simulink model "PthSet"  (R2018a)
settings: configuration reference "cs_ert" (kept outside this file)
settings Model: DataDictionary=PthSet.sldd  Creator=zhoutinglin  LastModifiedBy=zhoutinglin

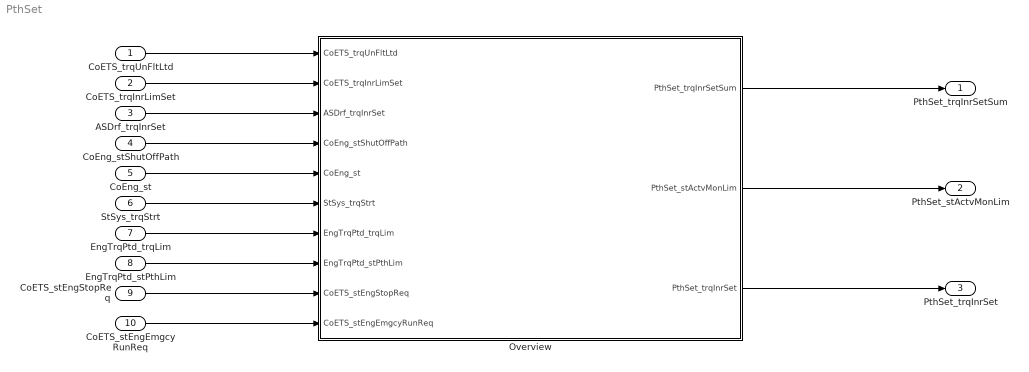
== system PthSet ==
  CoETS_trqUnFltLtd : Inport
  CoETS_trqInrLimSet : Inport  Port=2
  ASDrf_trqInrSet : Inport  Port=3
  CoEng_stShutOffPath : Inport  Port=4
  CoEng_st : Inport  Port=5
  StSys_trqStrt : Inport  Port=6
  EngTrqPtd_trqLim : Inport  Port=7
  EngTrqPtd_stPthLim : Inport  Port=8
  CoETS_stEngStopReq : Inport  Port=9
  CoETS_stEngEmgcyRunReq : Inport  Port=10
  Overview : Subsystem
  PthSet_trqInrSetSum : Outport
  PthSet_stActvMonLim : Outport  Port=2
  PthSet_trqInrSet : Outport  Port=3
  wires:
  CoETS_trqUnFltLtd/1 -> Overview/1(CoETS_trqUnFltLtd)
  CoETS_trqInrLimSet/1 -> Overview/2(CoETS_trqInrLimSet)
  ASDrf_trqInrSet/1 -> Overview/3(ASDrf_trqInrSet)
  CoEng_stShutOffPath/1 -> Overview/4(CoEng_stShutOffPath)
  CoEng_st/1 -> Overview/5(CoEng_st)
  StSys_trqStrt/1 -> Overview/6(StSys_trqStrt)
  EngTrqPtd_trqLim/1 -> Overview/7(EngTrqPtd_trqLim)
  EngTrqPtd_stPthLim/1 -> Overview/8(EngTrqPtd_stPthLim)
  CoETS_stEngStopReq/1 -> Overview/9(CoETS_stEngStopReq)
  CoETS_stEngEmgcyRunReq/1 -> Overview/10(CoETS_stEngEmgcyRunReq)
  Overview/1(PthSet_trqInrSetSum) -> PthSet_trqInrSetSum/1
  Overview/2(PthSet_stActvMonLim) -> PthSet_stActvMonLim/1
  Overview/3(PthSet_trqInrSet) -> PthSet_trqInrSet/1

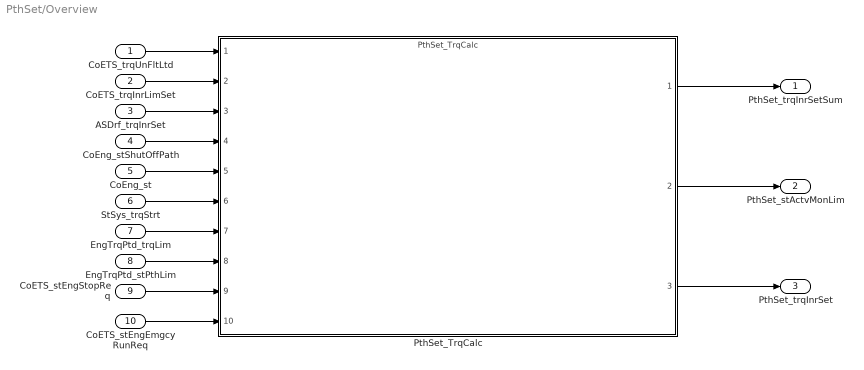
== system PthSet/Overview ==
  CoETS_trqUnFltLtd : Inport
  CoETS_trqInrLimSet : Inport  Port=2
  ASDrf_trqInrSet : Inport  Port=3
  CoEng_stShutOffPath : Inport  Port=4
  CoEng_st : Inport  Port=5
  StSys_trqStrt : Inport  Port=6
  EngTrqPtd_trqLim : Inport  Port=7
  EngTrqPtd_stPthLim : Inport  Port=8
  CoETS_stEngStopReq : Inport  Port=9
  CoETS_stEngEmgcyRunReq : Inport  Port=10
  PthSet_TrqCalc : ModelReference  ModelNameDialog=PthSet_TrqCalc  SimulationMode=Normal  ModelReferenceVersion=1.52
  PthSet_trqInrSetSum : Outport
  PthSet_stActvMonLim : Outport  Port=2
  PthSet_trqInrSet : Outport  Port=3
  wires:
  CoETS_trqUnFltLtd/1 -> PthSet_TrqCalc/1
  CoETS_trqInrLimSet/1 -> PthSet_TrqCalc/2
  ASDrf_trqInrSet/1 -> PthSet_TrqCalc/3
  CoEng_stShutOffPath/1 -> PthSet_TrqCalc/4
  CoEng_st/1 -> PthSet_TrqCalc/5
  StSys_trqStrt/1 -> PthSet_TrqCalc/6
  EngTrqPtd_trqLim/1 -> PthSet_TrqCalc/7
  EngTrqPtd_stPthLim/1 -> PthSet_TrqCalc/8
  CoETS_stEngStopReq/1 -> PthSet_TrqCalc/9
  CoETS_stEngEmgcyRunReq/1 -> PthSet_TrqCalc/10
  PthSet_TrqCalc/1 -> PthSet_trqInrSetSum/1
  PthSet_TrqCalc/2 -> PthSet_stActvMonLim/1
  PthSet_TrqCalc/3 -> PthSet_trqInrSet/1
